simulink model "model"  (R2023b)
settings: Solver=VariableStepAuto  StartTime=0.0  StopTime=10.0  RelTol=1e-3
undefined symbols (not defined in the file): DiscIntNeverNeededParam, Newton, Raphson
libraries: simulink x43, slpidlib x11
(part 2 of 2)

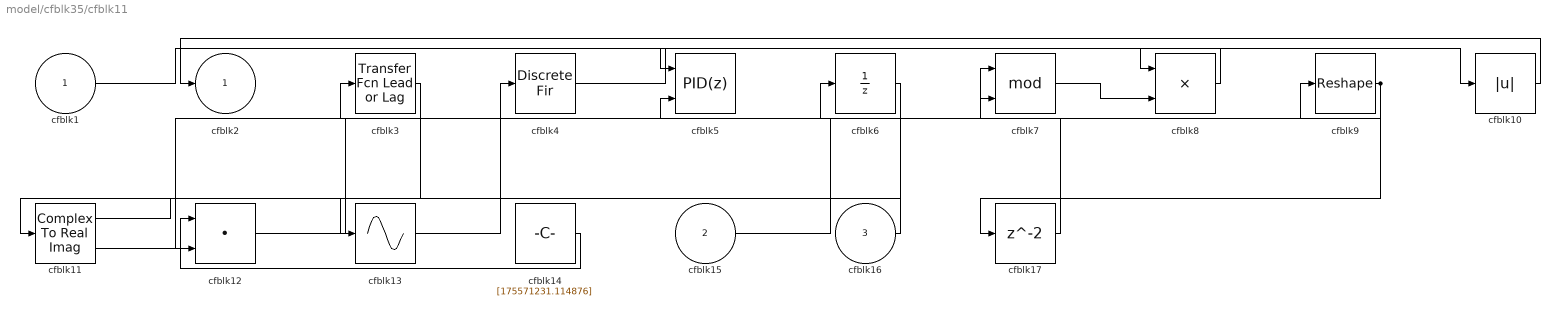
== system model/cfblk35/cfblk11 ==
  cfblk1 : Inport
  cfblk15 : Inport  Port=2
  cfblk16 : Inport  Port=3
  cfblk10 : Abs  SaturateOnIntegerOverflow=off
  cfblk11 : ComplexToRealImag
  cfblk12 : DotProduct  OutDataTypeStr=Inherit: Inherit via internal rule
  cfblk13 : Sin  TimeSource=Use external signal  SampleTime=0
  cfblk14 : Constant  Value=[175571231.114876]  SampleTime=1
  cfblk17 : Delay  SampleTime=1
  cfblk3 : simulink/Discrete/Transfer Fcn Lead or Lag  PoleZ=0.95  ZeroZ=0.75  ICPrevOutput=0.0  ICPrevInput=0.0  DoSatur=off
  cfblk4 : DiscreteFir  SampleTime=1
  cfblk5 : slpidlib/PID Controller (2DOF)  Controller=PID  Form=Parallel  TimeDomain=Discrete-time  UseExternalTs=off  SampleTime=1  IntegratorMethod=Forward Euler  FilterMethod=Forward Euler  ControllerParametersSource=internal  P=1  I=1  UseKiTs=off  D=0  N=100  UseFilter=on  b=1  c=1  TunerSelectOption=Transfer Function Based (PID Tuner App)  InitialConditionSource=internal  InitialConditionForIntegrator=0  InitialConditionForFilter=0  DifferentiatorICPrevScaledInput=0  ExternalReset=none  TrackingMode=off  Kt=1  LimitOutput=off  SatLimitsSource=internal  UpperSaturationLimit=inf  LowerSaturationLimit=-inf  LinearizeAsGain=off  AntiWindupMode=none  Kb=1  LimitIntegrator=off  UpperIntegratorSaturationLimit=inf  LowerIntegratorSaturationLimit=-inf  POutMin=[]  POutMax=[]  IOutMin=[]  IOutMax=[]  DOutMin=[]  DOutMax=[]  NOutMin=[]  NOutMax=[]  bOutMin=[]  bOutMax=[]  cOutMin=[]  cOutMax=[]  SumOutMin=[]  SumOutMax=[]  SaturationOutMin=[]  SaturationOutMax=[]  PParamMin=[]  PParamMax=[]  IParamMin=[]  IParamMax=[]  DParamMin=[]  DParamMax=[]  NParamMin=[]  NParamMax=[]  bParamMin=[]  bParamMax=[]  cParamMin=[]  cParamMax=[]  KbParamMin=[]  KbParamMax=[]  KtParamMin=[]  KtParamMax=[]  KbOutMin=[]  KbOutMax=[]  KtOutMin=[]  KtOutMax=[]  IntegratorOutMin=[]  IntegratorOutMax=[]  FilterOutMin=[]  FilterOutMax=[]  SumI1OutMin=[]  SumI1OutMax=[]  SumI2OutMin=[]  SumI2OutMax=[]  SumI3OutMin=[]  SumI3OutMax=[]  SumI4OutMin=[]  SumI4OutMax=[]  SumDOutMin=[]  SumDOutMax=[]  Sum1OutMin=[]  Sum1OutMax=[]  Sum2OutMin=[]  Sum2OutMax=[]  Sum3OutMin=[]  Sum3OutMax=[]  DifferentiatorOutMin=[]  DifferentiatorOutMax=[]  FilterDiffOutCoefMin=[]  FilterDiffOutCoefMax=[]  ReciprocalOutMin=[]  ReciprocalOutMax=[]  SumDenOutMin=[]  SumDenOutMax=[]  SumNumOutMin=[]  SumNumOutMax=[]  DivideOutMin=[]  DivideOutMax=[]  UdiffTsProdOutMin=[]  UdiffTsProdOutMax=[]  NTsProdOutMin=[]  NTsProdOutMax=[]  UintegralTsProdOutMin=[]  UintegralTsProdOutMax=[]  UngainTsProdOutMin=[]  UngainTsProdOutMax=[]  ClampingZeroOutDataTypeStr=Inherit: Inherit via back propagation  ClampingZeroOutMin=[]  ClampingZeroOutMax=[]  FilterDenConstantOutDataTypeStr=Inherit: Inherit via back propagation  FilterDenConstantOutMin=[]  FilterDenConstantOutMax=[]  PCopyOutDataTypeStr=Inherit: Inherit via back propagation  PCopyOutMin=[]  PCopyOutMax=[]  NCopyOutDataTypeStr=Inherit: Inherit via back propagation  NCopyOutMin=[]  NCopyOutMax=[]  IntegratorContinuousStateAttributes=''  IntegratorStateMustResolveToSignalObject=off  IntegratorRTWStateStorageClass=Auto  FilterContinuousStateAttributes=''  FilterStateMustResolveToSignalObject=off  FilterRTWStateStorageClass=Auto  ParallelPVariant=InternalParameters  IdealPVariant=Disabled  IVariant=InternalParameters  DVariant=InternalParameters  bVariant=InternalParameters  cVariant=InternalParameters  IntegratorVariant=Discrete  SatVariant=Disabled  AWVariant=Passthrough  PCopyVariant=Disabled  TRVariant=Disabled  FdbkBlocksVariant=Forward  IdealPFdbkVariant=Disabled  SatFdbkVariant=Disabled  DerivativeFilterVariant=ForwardEulerFilter  NVariant=InternalParameters  NCopyVariant=Disabled  FilterICVariant=InternalICsFilter  IntegratorICVariant=InternalICs  ExternalResetVariant=Disabled  TRSumVariant=Passthrough  SumFdbkVariant=Disabled  SumVariant=Sum_PID  TsampFilterVariant=InternalTs  TsampNgainVariant=Passthrough  TsampIntegralVariant=Disabled_SignalSpec  ExternalSaturationOutDataTypeStr=Inherit: Same as second input
      settings: LibrarySourceBlock=simulink/Discrete/Discrete PID Controller (2DOF)
  cfblk6 : UnitDelay  HasFrameUpgradeWarning=on
  cfblk7 : Math  Operator=mod
  cfblk8 : Product
  cfblk9 : Reshape
  cfblk2 : Outport
  wires:
  cfblk4/1 -> cfblk10/1
  cfblk9/1 -> cfblk5/2, cfblk17/1
  cfblk12/1 -> cfblk9/1
  cfblk16/1 -> cfblk6/1
  cfblk10/1 -> cfblk2/1
  cfblk14/1 -> cfblk12/1
  cfblk11/1 -> cfblk13/1
  cfblk3/1 -> cfblk12/2
  cfblk15/1 -> cfblk7/1
  cfblk6/1 -> cfblk11/1
  cfblk11/2 -> cfblk7/2
  cfblk1/1 -> cfblk8/1
  cfblk8/1 -> cfblk5/1
  cfblk7/1 -> cfblk8/2
  cfblk13/1 -> cfblk4/1
  cfblk17/1 -> cfblk3/1

== system model/cfblk36/cfblk10 ==
  cfblk1 : Inport
  cfblk10 : Delay  SampleTime=1
  cfblk3 : UnitDelay  HasFrameUpgradeWarning=on
  cfblk4 : DiscreteIntegrator  ICPrevOutput=DiscIntNeverNeededParam  ICPrevScaledInput=DiscIntNeverNeededParam
  cfblk5 : Polyval  Coefs=[ +2.081618890e-019, -1.441693666e-014, +4.719686976e-010, -8.536869453e-006, +1.621573104e-001, -8.087801117e+001 ]
  cfblk2 : Outport
  cfblk6 : Outport  Port=2
  cfblk7 : Outport  Port=3
  cfblk8 : Outport  Port=4
  cfblk9 : Outport  Port=5
  wires:
  cfblk1/1 -> cfblk7/1
  cfblk5/1 -> cfblk8/1, cfblk2/1, cfblk4/1, cfblk6/1
  cfblk3/1 -> cfblk9/1, cfblk5/1
  cfblk4/1 -> cfblk10/1
  cfblk10/1 -> cfblk3/1

== system model/cfblk36/cfblk11 ==
  cfblk1 : Inport
  cfblk12 : Inport  Port=2
  cfblk10 : Sqrt
  cfblk11 : Constant  Value=[-548459394.836145]  SampleTime=1
  cfblk14 : Delay  SampleTime=1
  cfblk3 : DiscreteFilter  SampleTime=1
  cfblk4 : Squeeze
  cfblk5 : simulink/Math Operations/Slider Gain  gain=1  low=0  high=2
  cfblk6 : Abs  SaturateOnIntegerOverflow=off
  cfblk7 : Product
  cfblk8 : Bias  Bias=[-249517717.832807]  SaturateOnIntegerOverflow=off
  cfblk9 : Sqrt
  cfblk2 : Outport
  cfblk13 : Outport  Port=2
  wires:
  cfblk11/1 -> cfblk8/1
  cfblk9/1 -> cfblk13/1
  cfblk3/1 -> cfblk7/1
  cfblk12/1 -> cfblk7/2
  cfblk6/1 -> cfblk5/1
  cfblk7/1 -> cfblk6/1
  cfblk10/1 -> cfblk2/1
  cfblk8/1 -> cfblk4/1
  cfblk1/1 -> cfblk10/1
  cfblk4/1 -> cfblk9/1
  cfblk5/1 -> cfblk14/1
  cfblk14/1 -> cfblk3/1

== system model/cfblk36/cfblk12 ==
  cfblk1 : Inport
  cfblk5 : Inport  Port=2
  cfblk6 : Inport  Port=3
  cfblk7 : Inport  Port=4
  cfblk8 : Inport  Port=5
  cfblk3 : ComplexToMagnitudeAngle
  cfblk4 : Sum  Inputs=|++
  cfblk2 : Outport
  wires:
  cfblk6/1 -> cfblk2/1
  cfblk5/1 -> cfblk3/1
  cfblk3/1 -> cfblk4/1
  cfblk7/1 -> cfblk4/2

== system model/cfblk37/cfblk10 ==
  cfblk1 : Inport
  cfblk13 : Inport  Port=2
  cfblk14 : Inport  Port=3
  cfblk15 : Inport  Port=4
  cfblk16 : Inport  Port=5
  cfblk10 : PermuteDimensions
  cfblk11 : Product  Inputs=*
  cfblk12 : Sum
  cfblk3 : simulink/Discrete/Tapped Delay  vinit=0.0  samptime=-1  NumDelays=1  DelayOrder=Oldest  includeCurrent=off
  cfblk4 : simulink/Discrete/Difference  ICPrevInput=0.0  OutMin=[]  OutMax=[]  OutDataTypeStr=Inherit: Inherit via back propagation  OutDataType=fixdt(1, 16)  OutScaling=2^-10  DoSatur=off
  cfblk5 : simulink/Discrete/Transfer Fcn First Order  PoleZ=0.95  ICPrevOutput=0.0  DoSatur=off
  cfblk6 : simulink/Discrete/Transfer Fcn Lead or Lag  PoleZ=0.95  ZeroZ=0.75  ICPrevOutput=0.0  ICPrevInput=0.0  DoSatur=off
  cfblk7 : Sum
  cfblk8 : Sum  Inputs=+-
  cfblk9 : simulink/Math Operations/Slider Gain  gain=1  low=0  high=2
  cfblk2 : Outport
  wires:
  cfblk15/1 -> cfblk5/1
  cfblk5/1 -> cfblk12/1
  cfblk4/1 -> cfblk2/1
  cfblk7/1 -> cfblk6/1
  cfblk13/1 -> cfblk7/1
  cfblk6/1 -> cfblk11/1
  cfblk11/1 -> cfblk3/1
  cfblk10/1 -> cfblk9/1
  cfblk9/1 -> cfblk7/2
  cfblk14/1 -> cfblk12/2
  cfblk12/1 -> cfblk10/1
  cfblk1/1 -> cfblk4/1
  cfblk16/1 -> cfblk8/1
  cfblk3/1 -> cfblk8/2

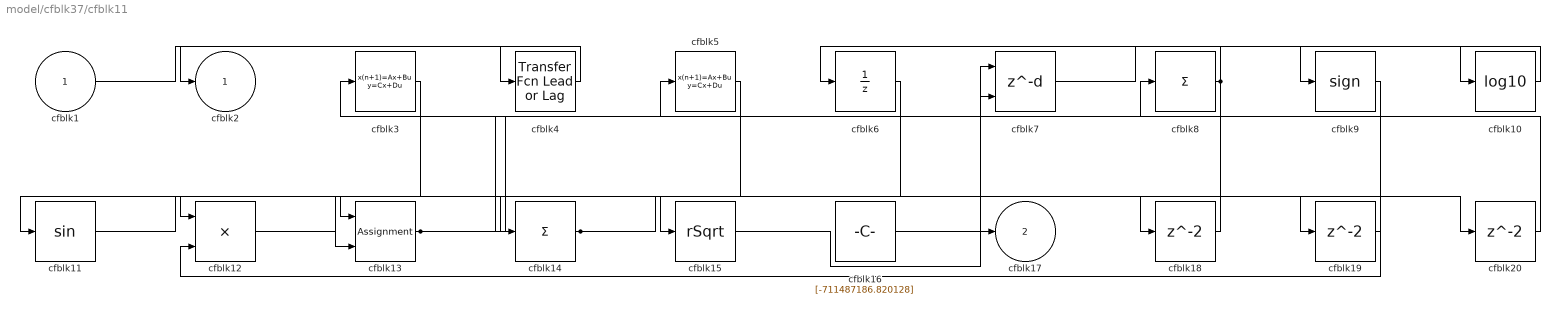
== system model/cfblk37/cfblk11 ==
  cfblk1 : Inport
  cfblk10 : Math  Operator=log10
  cfblk11 : Trigonometry
  cfblk12 : Product  Inputs=**
  cfblk13 : Assignment  DiagnosticForDimensions=Warning  IndexOptions=Index vector (dialog)  Indices=1  OutputSizes=1
  cfblk14 : Sum  Inputs=+
  cfblk15 : Sqrt  Operator=rSqrt  AlgorithmType=Newton-Raphson
  cfblk16 : Constant  Value=[-711487186.820128]  SampleTime=1
  cfblk18 : Delay  SampleTime=1
  cfblk19 : Delay  SampleTime=1
  cfblk20 : Delay  SampleTime=1
  cfblk3 : DiscreteStateSpace
  cfblk4 : simulink/Discrete/Transfer Fcn Lead or Lag  PoleZ=0.95  ZeroZ=0.75  ICPrevOutput=0.0  ICPrevInput=0.0  DoSatur=off
  cfblk5 : DiscreteStateSpace
  cfblk6 : UnitDelay  HasFrameUpgradeWarning=on
  cfblk7 : Delay  DelayLengthSource=Input port  SampleTime=1
      settings: InputPortMap=u0,p1
  cfblk8 : Sum  Inputs=+
  cfblk9 : Signum
  cfblk2 : Outport
  cfblk17 : Outport  Port=2
  wires:
  cfblk4/1 -> cfblk2/1
  cfblk6/1 -> cfblk11/1
  cfblk14/1 -> cfblk18/1, cfblk19/1
  cfblk15/1 -> cfblk7/1
  cfblk10/1 -> cfblk9/1
  cfblk16/1 -> cfblk17/1
  cfblk5/1 -> cfblk12/1
  cfblk9/1 -> cfblk12/2
  cfblk11/1 -> cfblk15/1
  cfblk1/1 -> cfblk4/1
  cfblk13/1 -> cfblk8/1, cfblk5/1
  cfblk8/1 -> cfblk14/1, cfblk6/1
  cfblk7/1 -> cfblk10/1
  cfblk3/1 -> cfblk13/2
  cfblk18/1 -> cfblk13/1
  cfblk19/1 -> cfblk3/1
  cfblk12/1 -> cfblk20/1
  cfblk20/1 -> cfblk7/2

== system model/cfblk37/cfblk12 ==
  cfblk1 : Inport
  cfblk16 : Inport  Port=2
  cfblk10 : Delay  SampleTime=1
  cfblk11 : DiscreteZeroPole  Poles=[0 0.5]  Gain=1
  cfblk12 : Sum  Inputs=-+
  cfblk13 : Sqrt  Operator=rSqrt  AlgorithmType=Newton-Raphson
  cfblk14 : UnaryMinus
  cfblk15 : Constant  Value=[60376909.899048]  SampleTime=1
  cfblk3 : simulink/Discrete/Tapped Delay  vinit=0.0  samptime=-1  NumDelays=1  DelayOrder=Oldest  includeCurrent=off
  cfblk4 : DiscreteStateSpace
  cfblk5 : UnitDelay  HasFrameUpgradeWarning=on
  cfblk6 : Delay  DelayLengthSource=Input port  SampleTime=1
      settings: InputPortMap=u0,p1
  cfblk7 : simulink/Discrete/Tapped Delay  vinit=0.0  samptime=-1  NumDelays=1  DelayOrder=Oldest  includeCurrent=off
  cfblk8 : DiscreteFir  SampleTime=1
  cfblk9 : DiscreteFir  SampleTime=1
  cfblk2 : Outport
  wires:
  cfblk10/1 -> cfblk9/1
  cfblk14/1 -> cfblk11/1
  cfblk7/1 -> cfblk14/1
  cfblk11/1 -> cfblk6/1
  cfblk1/1 -> cfblk3/1
  cfblk15/1 -> cfblk7/1
  cfblk6/1 -> cfblk5/1
  cfblk5/1 -> cfblk8/1
  cfblk16/1 -> cfblk13/1
  cfblk4/1 -> cfblk2/1
  cfblk9/1 -> cfblk12/1
  cfblk12/1 -> cfblk4/1
  cfblk8/1 -> cfblk12/2
  cfblk3/1 -> cfblk10/1
  cfblk13/1 -> cfblk6/2

== system model/cfblk37/cfblk13 ==
  cfblk1 : Inport
  cfblk11 : Inport  Port=2
  cfblk12 : Inport  Port=3
  cfblk13 : Inport  Port=4
  cfblk10 : Constant  Value=[801323161.151819]  SampleTime=1
  cfblk15 : Delay  SampleTime=1
  cfblk3 : PropagationDelay  SampleTime=1
  cfblk4 : Delay  ShowEnablePort=on  SampleTime=1
      settings: InputPortMap=u0,e6
  cfblk5 : simulink/Discrete/Transfer Fcn First Order  PoleZ=0.95  ICPrevOutput=0.0  DoSatur=off
  cfblk6 : UnitDelay  HasFrameUpgradeWarning=on
  cfblk7 : Signum
  cfblk8 : Squeeze
  cfblk9 : Sqrt  Operator=rSqrt  AlgorithmType=Newton-Raphson
  cfblk2 : Outport
  cfblk14 : Outport  Port=2
  wires:
  cfblk1/1 -> cfblk9/1
  cfblk3/1 -> cfblk7/1
  cfblk8/1 -> cfblk6/1
  cfblk10/1 -> cfblk4/1
  cfblk7/1 -> cfblk8/1
  cfblk4/1 -> cfblk2/1
  cfblk12/1 -> cfblk14/1
  cfblk11/1 -> cfblk5/1
  cfblk13/1 -> cfblk4/2
  cfblk9/1 -> cfblk3/1
  cfblk6/1 -> cfblk15/1
  cfblk15/1 -> cfblk3/2

== system model/cfblk37/cfblk8 ==
  cfblk1 : Inport
  cfblk9 : Inport  Port=2
  cfblk10 : Inport  Port=3
  cfblk11 : Delay  SampleTime=1
  cfblk3 : Delay  SampleTime=1
  cfblk4 : Product  Inputs=**
  cfblk5 : ComplexToMagnitudeAngle
  cfblk6 : Bias  Bias=[-189507740.076034]  SaturateOnIntegerOverflow=off
  cfblk7 : Squeeze
  cfblk8 : Constant  Value=[-524057900.089816]  SampleTime=1
  cfblk2 : Outport
  wires:
  cfblk4/1 -> cfblk7/1
  cfblk10/1 -> cfblk4/1
  cfblk9/1 -> cfblk6/1
  cfblk8/1 -> cfblk2/1
  cfblk6/1 -> cfblk5/1
  cfblk3/1 -> cfblk4/2
  cfblk7/1 -> cfblk11/1
  cfblk11/1 -> cfblk3/1

== system model/cfblk37/cfblk9 ==
  cfblk1 : Inport
  cfblk8 : Inport  Port=2
  cfblk9 : Inport  Port=3
  cfblk10 : Inport  Port=4
  cfblk11 : Inport  Port=5
  cfblk3 : DiscreteIntegrator  ICPrevOutput=DiscIntNeverNeededParam  ICPrevScaledInput=DiscIntNeverNeededParam
  cfblk4 : Product
  cfblk5 : Product  Inputs=*
  cfblk6 : Bias  Bias=[-689175598.464851]  SaturateOnIntegerOverflow=off
  cfblk7 : Sin  TimeSource=Use external signal  SampleTime=0
  cfblk2 : Outport
  cfblk12 : Outport  Port=2
  wires:
  cfblk9/1 -> cfblk3/1
  cfblk8/1 -> cfblk4/1
  cfblk5/1 -> cfblk6/1
  cfblk1/1 -> cfblk7/1
  cfblk11/1 -> cfblk4/2
  cfblk10/1 -> cfblk5/1
  cfblk4/1 -> cfblk2/1
  cfblk3/1 -> cfblk12/1

== system model/cfblk38/cfblk10 ==
  cfblk1 : Inport
  cfblk12 : Inport  Port=2
  cfblk13 : Inport  Port=3
  cfblk10 : MinMax  Inputs=2
  cfblk11 : Constant  Value=[-818087666.573941]  SampleTime=1
  cfblk3 : UnitDelay  HasFrameUpgradeWarning=on
  cfblk4 : Gain  Gain=[-630137339.256016]
  cfblk5 : Sum  Inputs=+
  cfblk6 : Sum  Inputs=+
  cfblk7 : Product  Inputs=*
  cfblk8 : Abs  SaturateOnIntegerOverflow=off
  cfblk9 : Reshape
  cfblk2 : Outport
  cfblk14 : Outport  Port=2
  wires:
  cfblk10/1 -> cfblk3/1
  cfblk3/1 -> cfblk8/1
  cfblk1/1 -> cfblk9/1
  cfblk8/1 -> cfblk5/1
  cfblk9/1 -> cfblk10/1
  cfblk11/1 -> cfblk6/1
  cfblk6/1 -> cfblk4/1
  cfblk4/1 -> cfblk10/2
  cfblk12/1 -> cfblk14/1
  cfblk5/1 -> cfblk7/1
  cfblk13/1 -> cfblk2/1

== system model/cfblk38/cfblk11 ==
  cfblk1 : Inport
  cfblk7 : Inport  Port=2
  cfblk3 : Delay  SampleTime=1
  cfblk4 : Delay  SampleTime=1
  cfblk5 : DiscreteFilter  SampleTime=1
  cfblk6 : Constant  Value=[-364935812.743680]  SampleTime=1
  cfblk2 : Outport
  cfblk8 : Outport  Port=2
  cfblk9 : Outport  Port=3
  wires:
  cfblk3/1 -> cfblk8/1
  cfblk1/1 -> cfblk5/1
  cfblk6/1 -> cfblk2/1
  cfblk5/1 -> cfblk4/1
  cfblk7/1 -> cfblk3/1
  cfblk4/1 -> cfblk9/1

== system model/cfblk38/cfblk12 ==
  cfblk1 : Inport
  cfblk3 : simulink/Discrete/Tapped Delay  vinit=0.0  samptime=-1  NumDelays=1  DelayOrder=Oldest  includeCurrent=off
  cfblk4 : Delay  ShowEnablePort=on  SampleTime=1
      settings: InputPortMap=u0,e6
  cfblk5 : DiscreteStateSpace
  cfblk6 : Gain  Gain=[600080903.886749]
  cfblk7 : Constant  Value=[-234072061.561648]  SampleTime=1
  cfblk8 : Constant  Value=[261940061.703511]  SampleTime=1
  cfblk2 : Outport
  wires:
  cfblk3/1 -> cfblk4/1
  cfblk7/1 -> cfblk3/1
  cfblk1/1 -> cfblk6/1
  cfblk5/1 -> cfblk4/2
  cfblk4/1 -> cfblk2/1
  cfblk6/1 -> cfblk5/1

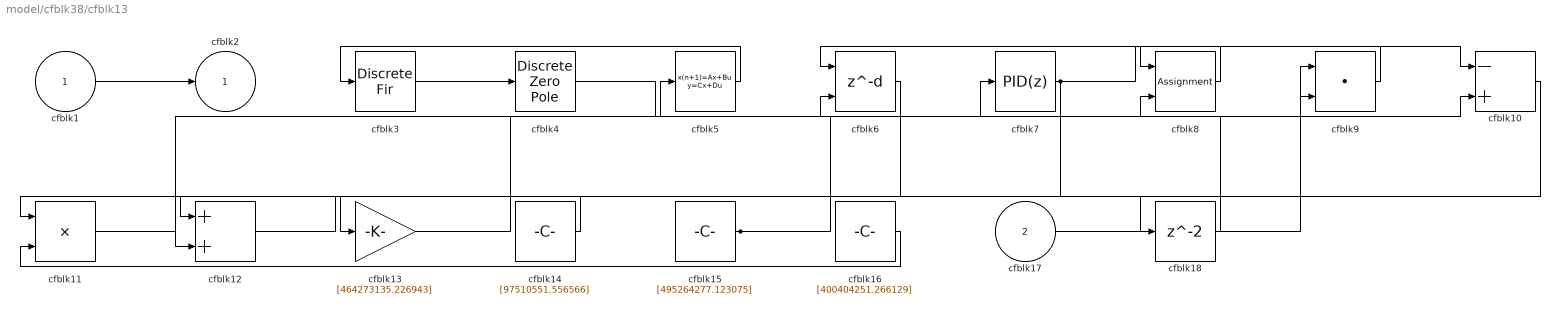
== system model/cfblk38/cfblk13 ==
  cfblk1 : Inport
  cfblk17 : Inport  Port=2
  cfblk10 : Sum  Inputs=-+
  cfblk11 : Product
  cfblk12 : Sum
  cfblk13 : Gain  Gain=[464273135.226943]
  cfblk14 : Constant  Value=[97510551.556566]  SampleTime=1
  cfblk15 : Constant  Value=[495264277.123075]  SampleTime=1
  cfblk16 : Constant  Value=[400404251.266129]  SampleTime=1
  cfblk18 : Delay  SampleTime=1
  cfblk3 : DiscreteFir  SampleTime=1
  cfblk4 : DiscreteZeroPole  Poles=[0 0.5]  Gain=1
  cfblk5 : DiscreteStateSpace
  cfblk6 : Delay  DelayLengthSource=Input port  SampleTime=1
      settings: InputPortMap=u0,p1
  cfblk7 : slpidlib/PID Controller  Controller=PID  Form=Parallel  TimeDomain=Discrete-time  UseExternalTs=off  SampleTime=1  IntegratorMethod=Forward Euler  FilterMethod=Forward Euler  ControllerParametersSource=internal  P=1  I=1  UseKiTs=off  D=0  N=100  UseFilter=on  TunerSelectOption=Transfer Function Based (PID Tuner App)  InitialConditionSource=internal  InitialConditionForIntegrator=0  InitialConditionForFilter=0  DifferentiatorICPrevScaledInput=0  ExternalReset=none  TrackingMode=off  Kt=1  LimitOutput=off  SatLimitsSource=internal  UpperSaturationLimit=inf  LowerSaturationLimit=-inf  LinearizeAsGain=off  AntiWindupMode=none  Kb=1  LimitIntegrator=off  UpperIntegratorSaturationLimit=inf  LowerIntegratorSaturationLimit=-inf  POutMin=[]  POutMax=[]  IOutMin=[]  IOutMax=[]  DOutMin=[]  DOutMax=[]  NOutMin=[]  NOutMax=[]  SumOutMin=[]  SumOutMax=[]  SaturationOutMin=[]  SaturationOutMax=[]  PParamMin=[]  PParamMax=[]  IParamMin=[]  IParamMax=[]  DParamMin=[]  DParamMax=[]  NParamMin=[]  NParamMax=[]  KbParamMin=[]  KbParamMax=[]  KtParamMin=[]  KtParamMax=[]  KbOutMin=[]  KbOutMax=[]  KtOutMin=[]  KtOutMax=[]  IntegratorOutMin=[]  IntegratorOutMax=[]  FilterOutMin=[]  FilterOutMax=[]  SumI1OutMin=[]  SumI1OutMax=[]  SumI2OutMin=[]  SumI2OutMax=[]  SumI3OutMin=[]  SumI3OutMax=[]  SumI4OutMin=[]  SumI4OutMax=[]  SumDOutMin=[]  SumDOutMax=[]  DifferentiatorOutMin=[]  DifferentiatorOutMax=[]  FilterDiffOutCoefMin=[]  FilterDiffOutCoefMax=[]  ReciprocalOutMin=[]  ReciprocalOutMax=[]  SumDenOutMin=[]  SumDenOutMax=[]  SumNumOutMin=[]  SumNumOutMax=[]  DivideOutMin=[]  DivideOutMax=[]  UdiffTsProdOutMin=[]  UdiffTsProdOutMax=[]  NTsProdOutMin=[]  NTsProdOutMax=[]  UintegralTsProdOutMin=[]  UintegralTsProdOutMax=[]  UngainTsProdOutMin=[]  UngainTsProdOutMax=[]  ClampingZeroOutDataTypeStr=Inherit: Inherit via back propagation  ClampingZeroOutMin=[]  ClampingZeroOutMax=[]  FilterDenConstantOutDataTypeStr=Inherit: Inherit via back propagation  FilterDenConstantOutMin=[]  FilterDenConstantOutMax=[]  PCopyOutDataTypeStr=Inherit: Inherit via back propagation  PCopyOutMin=[]  PCopyOutMax=[]  NCopyOutDataTypeStr=Inherit: Inherit via back propagation  NCopyOutMin=[]  NCopyOutMax=[]  IntegratorContinuousStateAttributes=''  IntegratorStateMustResolveToSignalObject=off  IntegratorRTWStateStorageClass=Auto  FilterContinuousStateAttributes=''  FilterStateMustResolveToSignalObject=off  FilterRTWStateStorageClass=Auto  ParallelPVariant=InternalParameters  IdealPVariant=Disabled  IVariant=InternalParameters  DVariant=InternalParameters  IntegratorVariant=Discrete  SatVariant=Disabled  AWVariant=Passthrough  PCopyVariant=Disabled  TRVariant=Disabled  FdbkBlocksVariant=Forward  IdealPFdbkVariant=Disabled  SatFdbkVariant=Disabled  DerivativeFilterVariant=ForwardEulerFilter  NVariant=InternalParameters  NCopyVariant=Disabled  FilterICVariant=InternalICsFilter  IntegratorICVariant=InternalICs  ExternalResetVariant=Disabled  TRSumVariant=Passthrough  SumFdbkVariant=Disabled  SumVariant=Sum_PID  TsampFilterVariant=InternalTs  TsampNgainVariant=Passthrough  TsampIntegralVariant=Disabled_SignalSpec  ExternalSaturationOutDataTypeStr=Inherit: Same as second input
      settings: LibrarySourceBlock=simulink/Discrete/Discrete PID Controller
  cfblk8 : Assignment  DiagnosticForDimensions=Warning  IndexOptions=Index vector (dialog)  Indices=1  OutputSizes=1
  cfblk9 : DotProduct  OutDataTypeStr=Inherit: Inherit via internal rule
  cfblk2 : Outport
  wires:
  cfblk1/1 -> cfblk2/1
  cfblk10/1 -> cfblk11/1
  cfblk16/1 -> cfblk11/2
  cfblk14/1 -> cfblk13/1
  cfblk3/1 -> cfblk4/1
  cfblk9/1 -> cfblk8/1
  cfblk6/1 -> cfblk12/1
  cfblk5/1 -> cfblk3/1
  cfblk13/1 -> cfblk5/1
  cfblk17/1 -> cfblk9/1
  cfblk15/1 -> cfblk7/1, cfblk10/2
  cfblk11/1 -> cfblk8/2
  cfblk8/1 -> cfblk6/1
  cfblk7/1 -> cfblk12/2, cfblk10/1
  cfblk4/1 -> cfblk9/2
  cfblk12/1 -> cfblk18/1
  cfblk18/1 -> cfblk6/2

== system model/cfblk38/cfblk14 ==
  cfblk1 : Inport
  cfblk14 : Inport  Port=2
  cfblk15 : Inport  Port=3
  cfblk10 : Squeeze
  cfblk11 : PermuteDimensions
  cfblk12 : Product  Inputs=*
  cfblk13 : Sqrt
  cfblk3 : UnitDelay  HasFrameUpgradeWarning=on
  cfblk4 : slpidlib/PID Controller  Controller=PID  Form=Parallel  TimeDomain=Discrete-time  UseExternalTs=off  SampleTime=1  IntegratorMethod=Forward Euler  FilterMethod=Forward Euler  ControllerParametersSource=internal  P=1  I=1  UseKiTs=off  D=0  N=100  UseFilter=on  TunerSelectOption=Transfer Function Based (PID Tuner App)  InitialConditionSource=internal  InitialConditionForIntegrator=0  InitialConditionForFilter=0  DifferentiatorICPrevScaledInput=0  ExternalReset=none  TrackingMode=off  Kt=1  LimitOutput=off  SatLimitsSource=internal  UpperSaturationLimit=inf  LowerSaturationLimit=-inf  LinearizeAsGain=off  AntiWindupMode=none  Kb=1  LimitIntegrator=off  UpperIntegratorSaturationLimit=inf  LowerIntegratorSaturationLimit=-inf  POutMin=[]  POutMax=[]  IOutMin=[]  IOutMax=[]  DOutMin=[]  DOutMax=[]  NOutMin=[]  NOutMax=[]  SumOutMin=[]  SumOutMax=[]  SaturationOutMin=[]  SaturationOutMax=[]  PParamMin=[]  PParamMax=[]  IParamMin=[]  IParamMax=[]  DParamMin=[]  DParamMax=[]  NParamMin=[]  NParamMax=[]  KbParamMin=[]  KbParamMax=[]  KtParamMin=[]  KtParamMax=[]  KbOutMin=[]  KbOutMax=[]  KtOutMin=[]  KtOutMax=[]  IntegratorOutMin=[]  IntegratorOutMax=[]  FilterOutMin=[]  FilterOutMax=[]  SumI1OutMin=[]  SumI1OutMax=[]  SumI2OutMin=[]  SumI2OutMax=[]  SumI3OutMin=[]  SumI3OutMax=[]  SumI4OutMin=[]  SumI4OutMax=[]  SumDOutMin=[]  SumDOutMax=[]  DifferentiatorOutMin=[]  DifferentiatorOutMax=[]  FilterDiffOutCoefMin=[]  FilterDiffOutCoefMax=[]  ReciprocalOutMin=[]  ReciprocalOutMax=[]  SumDenOutMin=[]  SumDenOutMax=[]  SumNumOutMin=[]  SumNumOutMax=[]  DivideOutMin=[]  DivideOutMax=[]  UdiffTsProdOutMin=[]  UdiffTsProdOutMax=[]  NTsProdOutMin=[]  NTsProdOutMax=[]  UintegralTsProdOutMin=[]  UintegralTsProdOutMax=[]  UngainTsProdOutMin=[]  UngainTsProdOutMax=[]  ClampingZeroOutDataTypeStr=Inherit: Inherit via back propagation  ClampingZeroOutMin=[]  ClampingZeroOutMax=[]  FilterDenConstantOutDataTypeStr=Inherit: Inherit via back propagation  FilterDenConstantOutMin=[]  FilterDenConstantOutMax=[]  PCopyOutDataTypeStr=Inherit: Inherit via back propagation  PCopyOutMin=[]  PCopyOutMax=[]  NCopyOutDataTypeStr=Inherit: Inherit via back propagation  NCopyOutMin=[]  NCopyOutMax=[]  IntegratorContinuousStateAttributes=''  IntegratorStateMustResolveToSignalObject=off  IntegratorRTWStateStorageClass=Auto  FilterContinuousStateAttributes=''  FilterStateMustResolveToSignalObject=off  FilterRTWStateStorageClass=Auto  ParallelPVariant=InternalParameters  IdealPVariant=Disabled  IVariant=InternalParameters  DVariant=InternalParameters  IntegratorVariant=Discrete  SatVariant=Disabled  AWVariant=Passthrough  PCopyVariant=Disabled  TRVariant=Disabled  FdbkBlocksVariant=Forward  IdealPFdbkVariant=Disabled  SatFdbkVariant=Disabled  DerivativeFilterVariant=ForwardEulerFilter  NVariant=InternalParameters  NCopyVariant=Disabled  FilterICVariant=InternalICsFilter  IntegratorICVariant=InternalICs  ExternalResetVariant=Disabled  TRSumVariant=Passthrough  SumFdbkVariant=Disabled  SumVariant=Sum_PID  TsampFilterVariant=InternalTs  TsampNgainVariant=Passthrough  TsampIntegralVariant=Disabled_SignalSpec  ExternalSaturationOutDataTypeStr=Inherit: Same as second input
      settings: LibrarySourceBlock=simulink/Discrete/Discrete PID Controller
  cfblk5 : simulink/Discrete/Tapped Delay  vinit=0.0  samptime=-1  NumDelays=1  DelayOrder=Oldest  includeCurrent=off
  cfblk6 : Sqrt
  cfblk7 : Assignment  DiagnosticForDimensions=Warning  IndexOptions=Index vector (dialog)  Indices=1  OutputSizes=1
  cfblk8 : Sin  TimeSource=Use external signal  SampleTime=0
  cfblk9 : Sin  TimeSource=Use external signal  SampleTime=0
  cfblk2 : Outport
  wires:
  cfblk4/1 -> cfblk12/1
  cfblk6/1 -> cfblk3/1
  cfblk1/1 -> cfblk5/1
  cfblk10/1 -> cfblk9/1
  cfblk11/1 -> cfblk10/1
  cfblk13/1 -> cfblk2/1
  cfblk15/1 -> cfblk4/1
  cfblk3/1 -> cfblk8/1
  cfblk5/1 -> cfblk6/1
  cfblk9/1 -> cfblk7/1
  cfblk14/1 -> cfblk11/1
  cfblk12/1 -> cfblk7/2
  cfblk7/1 -> cfblk13/1

== system model/cfblk38/cfblk8 ==
  cfblk1 : Inport
  cfblk9 : Inport  Port=2
  cfblk3 : Gain  Gain=[-893617306.951323]
  cfblk4 : Product
  cfblk5 : Sum  Inputs=+
  cfblk6 : Reshape
  cfblk7 : Trigonometry
  cfblk8 : Constant  Value=[719142667.653618]  SampleTime=1
  cfblk2 : Outport
  cfblk10 : Outport  Port=2
  cfblk11 : Outport  Port=3
  wires:
  cfblk5/1 -> cfblk3/1
  cfblk3/1 -> cfblk11/1
  cfblk8/1 -> cfblk4/1, cfblk7/1
  cfblk6/1 -> cfblk2/1
  cfblk9/1 -> cfblk4/2
  cfblk4/1 -> cfblk10/1
  cfblk1/1 -> cfblk5/1
  cfblk7/1 -> cfblk6/1

== system model/cfblk38/cfblk9 ==
  cfblk1 : Inport
  cfblk7 : Inport  Port=2
  cfblk8 : Inport  Port=3
  cfblk3 : DiscreteTransferFcn  SampleTime=1
  cfblk4 : UnaryMinus
  cfblk5 : UnaryMinus
  cfblk6 : Constant  Value=[970426307.203716]  SampleTime=1
  cfblk2 : Outport
  cfblk9 : Outport  Port=2
  cfblk10 : Outport  Port=3
  wires:
  cfblk5/1 -> cfblk2/1
  cfblk1/1 -> cfblk4/1
  cfblk7/1 -> cfblk3/1
  cfblk3/1 -> cfblk9/1
  cfblk6/1 -> cfblk5/1
  cfblk4/1 -> cfblk10/1

== system model/cfblk39/cfblk10 ==
  cfblk1 : Inport
  cfblk11 : Inport  Port=2
  cfblk12 : Inport  Port=3
  cfblk10 : Constant  Value=[-430199746.707510]  SampleTime=1
  cfblk3 : Delay  DelayLengthSource=Input port  SampleTime=1
      settings: InputPortMap=u0,p1
  cfblk4 : Sin  TimeSource=Use external signal  SampleTime=0
  cfblk5 : Sum  Inputs=+
  cfblk6 : PermuteDimensions
  cfblk7 : Sum  Inputs=|++
  cfblk8 : Product  Inputs=**
  cfblk9 : Sum  Inputs=+-
  cfblk2 : Outport
  cfblk13 : Outport  Port=2
  wires:
  cfblk10/1 -> cfblk6/1
  cfblk3/1 -> cfblk8/1
  cfblk5/1 -> cfblk4/1
  cfblk6/1 -> cfblk7/1, cfblk3/2
  cfblk8/1 -> cfblk13/1
  cfblk4/1 -> cfblk8/2
  cfblk1/1 -> cfblk7/2
  cfblk12/1 -> cfblk2/1, cfblk9/2
  cfblk11/1 -> cfblk5/1
  cfblk7/1 -> cfblk9/1
  cfblk9/1 -> cfblk3/1

== system model/cfblk39/cfblk11 ==
  cfblk1 : Inport
  cfblk9 : Inport  Port=2
  cfblk10 : Inport  Port=3
  cfblk11 : Inport  Port=4
  cfblk12 : Inport  Port=5
  cfblk3 : DiscreteStateSpace
  cfblk4 : DiscreteIntegrator  ICPrevOutput=DiscIntNeverNeededParam  ICPrevScaledInput=DiscIntNeverNeededParam
  cfblk5 : Sin  TimeSource=Use external signal  SampleTime=0
  cfblk6 : DotProduct  OutDataTypeStr=Inherit: Inherit via internal rule
  cfblk7 : Constant  Value=[-722446577.434283]  SampleTime=1
  cfblk8 : Constant  Value=[-47518749.440726]  SampleTime=1
  cfblk2 : Outport
  cfblk13 : Outport  Port=2
  cfblk14 : Outport  Port=3
  wires:
  cfblk9/1 -> cfblk6/1
  cfblk5/1 -> cfblk14/1
  cfblk11/1 -> cfblk4/1
  cfblk1/1 -> cfblk2/1
  cfblk10/1 -> cfblk6/2
  cfblk8/1 -> cfblk3/1
  cfblk7/1 -> cfblk5/1
  cfblk3/1 -> cfblk13/1

== system model/cfblk39/cfblk12 ==
  cfblk1 : Inport
  cfblk10 : Inport  Port=2
  cfblk11 : Inport  Port=3
  cfblk12 : Inport  Port=4
  cfblk14 : Delay  SampleTime=1
  cfblk3 : simulink/Discrete/Difference  ICPrevInput=0.0  OutMin=[]  OutMax=[]  OutDataTypeStr=Inherit: Inherit via back propagation  OutDataType=fixdt(1, 16)  OutScaling=2^-10  DoSatur=off
  cfblk4 : DiscreteZeroPole  Poles=[0 0.5]  Gain=1
  cfblk5 : Delay  ShowEnablePort=on  SampleTime=1
      settings: InputPortMap=u0,e6
  cfblk6 : Gain  Gain=[-375453854.574921]
  cfblk7 : Abs  SaturateOnIntegerOverflow=off
  cfblk8 : Constant  Value=[309716630.147981]  SampleTime=1
  cfblk9 : Constant  Value=[-168676981.693167]  SampleTime=1
  cfblk2 : Outport
  cfblk13 : Outport  Port=2
  wires:
  cfblk1/1 -> cfblk13/1
  cfblk8/1 -> cfblk4/1
  cfblk5/1 -> cfblk6/1
  cfblk10/1 -> cfblk7/1
  cfblk11/1 -> cfblk2/1
  cfblk7/1 -> cfblk5/1
  cfblk3/1 -> cfblk5/2
  cfblk6/1 -> cfblk14/1
  cfblk14/1 -> cfblk3/1

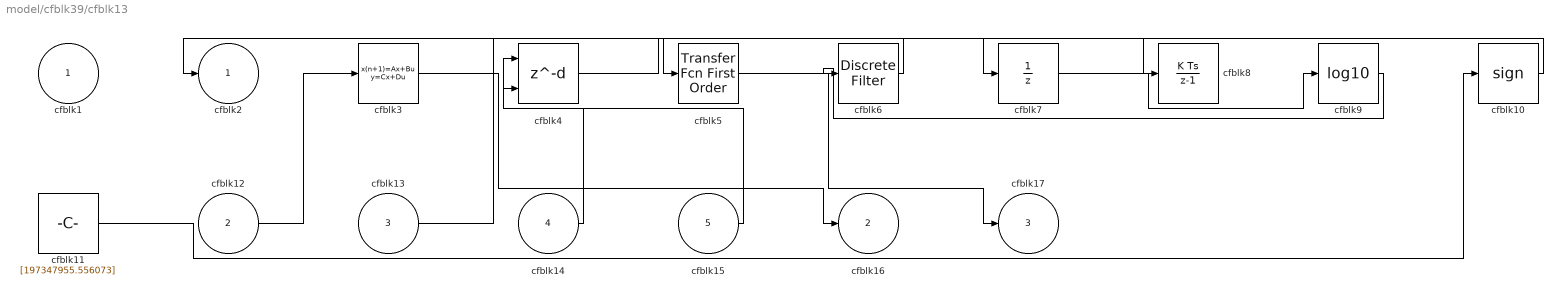
== system model/cfblk39/cfblk13 ==
  cfblk1 : Inport
  cfblk12 : Inport  Port=2
  cfblk13 : Inport  Port=3
  cfblk14 : Inport  Port=4
  cfblk15 : Inport  Port=5
  cfblk10 : Signum
  cfblk11 : Constant  Value=[197347955.556073]  SampleTime=1
  cfblk3 : DiscreteStateSpace
  cfblk4 : Delay  DelayLengthSource=Input port  SampleTime=1
      settings: InputPortMap=u0,p1
  cfblk5 : simulink/Discrete/Transfer Fcn First Order  PoleZ=0.95  ICPrevOutput=0.0  DoSatur=off
  cfblk6 : DiscreteFilter  SampleTime=1
  cfblk7 : UnitDelay  HasFrameUpgradeWarning=on
  cfblk8 : DiscreteIntegrator  ICPrevOutput=DiscIntNeverNeededParam  ICPrevScaledInput=DiscIntNeverNeededParam
  cfblk9 : Math  Operator=log10
  cfblk2 : Outport
  cfblk16 : Outport  Port=2
  cfblk17 : Outport  Port=3
  wires:
  cfblk12/1 -> cfblk3/1
  cfblk15/1 -> cfblk4/1
  cfblk5/1 -> cfblk17/1
  cfblk14/1 -> cfblk4/2
  cfblk10/1 -> cfblk7/1
  cfblk7/1 -> cfblk9/1
  cfblk13/1 -> cfblk5/1
  cfblk3/1 -> cfblk16/1
  cfblk4/1 -> cfblk8/1
  cfblk9/1 -> cfblk6/1
  cfblk6/1 -> cfblk2/1
  cfblk11/1 -> cfblk10/1

== system model/cfblk39/cfblk14 ==
  cfblk1 : Inport
  cfblk8 : Inport  Port=2
  cfblk9 : Inport  Port=3
  cfblk10 : Inport  Port=4
  cfblk3 : simulink/Discrete/Tapped Delay  vinit=0.0  samptime=-1  NumDelays=1  DelayOrder=Oldest  includeCurrent=off
  cfblk4 : Product  Inputs=**
  cfblk5 : Constant  Value=[-298102019.536058]  SampleTime=1
  cfblk6 : Constant  Value=[394898119.156315]  SampleTime=1
  cfblk7 : Constant  Value=[-946998443.364874]  SampleTime=1
  cfblk2 : Outport
  cfblk11 : Outport  Port=2
  wires:
  cfblk3/1 -> cfblk4/1
  cfblk8/1 -> cfblk2/1
  cfblk5/1 -> cfblk11/1
  cfblk1/1 -> cfblk4/2
  cfblk7/1 -> cfblk3/1

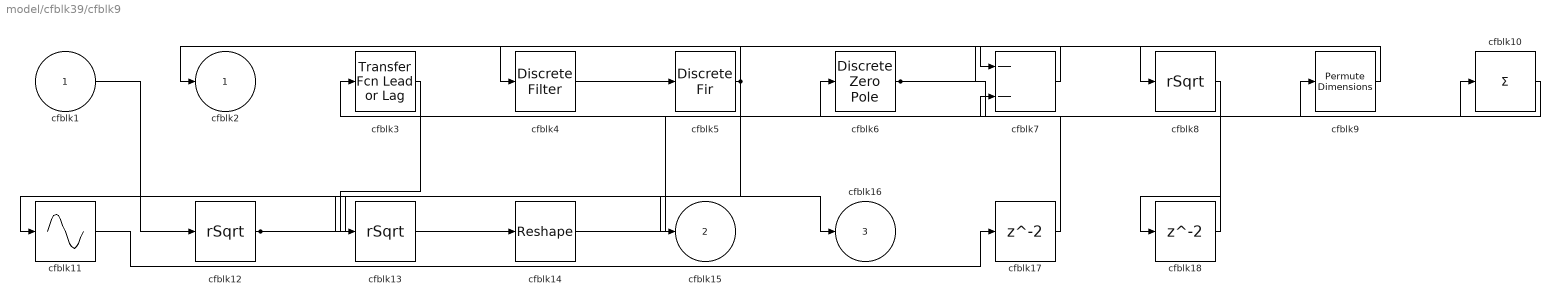
== system model/cfblk39/cfblk9 ==
  cfblk1 : Inport
  cfblk10 : Sum  Inputs=+
  cfblk11 : Sin  TimeSource=Use external signal  SampleTime=0
  cfblk12 : Sqrt  Operator=rSqrt  AlgorithmType=Newton-Raphson
  cfblk13 : Sqrt  Operator=rSqrt  AlgorithmType=Newton-Raphson
  cfblk14 : Reshape
  cfblk17 : Delay  SampleTime=1
  cfblk18 : Delay  SampleTime=1
  cfblk3 : simulink/Discrete/Transfer Fcn Lead or Lag  PoleZ=0.95  ZeroZ=0.75  ICPrevOutput=0.0  ICPrevInput=0.0  DoSatur=off
  cfblk4 : DiscreteFilter  SampleTime=1
  cfblk5 : DiscreteFir  SampleTime=1
  cfblk6 : DiscreteZeroPole  Poles=[0 0.5]  Gain=1
  cfblk7 : Sum  Inputs=--
  cfblk8 : Sqrt  Operator=rSqrt  AlgorithmType=Newton-Raphson
  cfblk9 : PermuteDimensions
  cfblk2 : Outport
  cfblk15 : Outport  Port=2
  cfblk16 : Outport  Port=3
  wires:
  cfblk9/1 -> cfblk7/1
  cfblk12/1 -> cfblk16/1, cfblk15/1
  cfblk5/1 -> cfblk2/1, cfblk11/1
  cfblk3/1 -> cfblk13/1
  cfblk13/1 -> cfblk14/1
  cfblk6/1 -> cfblk9/1, cfblk8/1
  cfblk4/1 -> cfblk5/1
  cfblk10/1 -> cfblk7/2
  cfblk1/1 -> cfblk12/1
  cfblk14/1 -> cfblk10/1
  cfblk7/1 -> cfblk4/1
  cfblk11/1 -> cfblk17/1
  cfblk17/1 -> cfblk3/1
  cfblk8/1 -> cfblk18/1
  cfblk18/1 -> cfblk6/1

== system model/cfblk40/cfblk11 ==
  cfblk1 : Inport
  Action Port : ActionPort  ActionPortLabel=if(u1 >= 0)
  cfblk10 : Constant  Value=[-596403052.275177]  SampleTime=1
  cfblk12 : Delay
  cfblk3 : DiscreteZeroPole  Poles=[0 0.5]  Gain=1  SampleTime=-1
  cfblk4 : DiscreteTransferFcn
  cfblk5 : DiscreteTransferFcn
  cfblk6 : Sum
  cfblk7 : UnaryMinus
  cfblk8 : Sum  Inputs=|++
  cfblk9 : MinMax  Function=max  Inputs=3
  cfblk2 : Outport
  cfblk11 : Outport  Port=2
  wires:
  cfblk3/1 -> cfblk9/1
  cfblk7/1 -> cfblk5/1
  cfblk5/1 -> cfblk4/1, cfblk3/1
  cfblk6/1 -> cfblk9/2, cfblk2/1
  cfblk8/1 -> cfblk6/2
  cfblk10/1 -> cfblk7/1
  cfblk4/1 -> cfblk8/1, cfblk11/1, cfblk9/3
  cfblk1/1 -> cfblk8/2
  cfblk9/1 -> cfblk12/1
  cfblk12/1 -> cfblk6/1

== system model/cfblk40/cfblk12 ==
  cfblk1 : Inport
  cfblk5 : Inport  Port=2
  Action Port : ActionPort  ActionPortLabel=else
  cfblk3 : Product  Inputs=**
  cfblk4 : Sum  Inputs=+
  cfblk2 : Outport
  cfblk6 : Outport  Port=2
  cfblk7 : Outport  Port=3
  wires:
  cfblk4/1 -> cfblk7/1, cfblk3/1
  cfblk1/1 -> cfblk4/1, cfblk3/2
  cfblk5/1 -> cfblk2/1
  cfblk3/1 -> cfblk6/1

== system model/cfblk40/cfblk6 ==
  cfblk1 : Inport
  cfblk5 : Inport  Port=2
  cfblk6 : Inport  Port=3
  cfblk3 : ComplexToMagnitudeAngle
  cfblk4 : Constant  Value=[953994063.598649]  SampleTime=1
  cfblk2 : Outport
  cfblk7 : Outport  Port=2
  cfblk8 : Outport  Port=3
  wires:
  cfblk5/1 -> cfblk3/1
  cfblk4/1 -> cfblk8/1
  cfblk1/1 -> cfblk7/1
  cfblk6/1 -> cfblk2/1

== system model/cfblk40/cfblk7 ==
  cfblk1 : Inport
  cfblk12 : Inport  Port=2
  cfblk13 : Inport  Port=3
  cfblk10 : Signum
  cfblk11 : Constant  Value=[242620350.389675]  SampleTime=1
  cfblk3 : simulink/Discrete/Transfer Fcn First Order  PoleZ=0.95  ICPrevOutput=0.0  DoSatur=off
  cfblk4 : simulink/Discrete/Transfer Fcn First Order  PoleZ=0.95  ICPrevOutput=0.0  DoSatur=off
  cfblk5 : DiscreteFilter  SampleTime=1
  cfblk6 : slpidlib/PID Controller  Controller=PID  Form=Parallel  TimeDomain=Discrete-time  UseExternalTs=off  SampleTime=1  IntegratorMethod=Forward Euler  FilterMethod=Forward Euler  ControllerParametersSource=internal  P=1  I=1  UseKiTs=off  D=0  N=100  UseFilter=on  TunerSelectOption=Transfer Function Based (PID Tuner App)  InitialConditionSource=internal  InitialConditionForIntegrator=0  InitialConditionForFilter=0  DifferentiatorICPrevScaledInput=0  ExternalReset=none  TrackingMode=off  Kt=1  LimitOutput=off  SatLimitsSource=internal  UpperSaturationLimit=inf  LowerSaturationLimit=-inf  LinearizeAsGain=off  AntiWindupMode=none  Kb=1  LimitIntegrator=off  UpperIntegratorSaturationLimit=inf  LowerIntegratorSaturationLimit=-inf  POutMin=[]  POutMax=[]  IOutMin=[]  IOutMax=[]  DOutMin=[]  DOutMax=[]  NOutMin=[]  NOutMax=[]  SumOutMin=[]  SumOutMax=[]  SaturationOutMin=[]  SaturationOutMax=[]  PParamMin=[]  PParamMax=[]  IParamMin=[]  IParamMax=[]  DParamMin=[]  DParamMax=[]  NParamMin=[]  NParamMax=[]  KbParamMin=[]  KbParamMax=[]  KtParamMin=[]  KtParamMax=[]  KbOutMin=[]  KbOutMax=[]  KtOutMin=[]  KtOutMax=[]  IntegratorOutMin=[]  IntegratorOutMax=[]  FilterOutMin=[]  FilterOutMax=[]  SumI1OutMin=[]  SumI1OutMax=[]  SumI2OutMin=[]  SumI2OutMax=[]  SumI3OutMin=[]  SumI3OutMax=[]  SumI4OutMin=[]  SumI4OutMax=[]  SumDOutMin=[]  SumDOutMax=[]  DifferentiatorOutMin=[]  DifferentiatorOutMax=[]  FilterDiffOutCoefMin=[]  FilterDiffOutCoefMax=[]  ReciprocalOutMin=[]  ReciprocalOutMax=[]  SumDenOutMin=[]  SumDenOutMax=[]  SumNumOutMin=[]  SumNumOutMax=[]  DivideOutMin=[]  DivideOutMax=[]  UdiffTsProdOutMin=[]  UdiffTsProdOutMax=[]  NTsProdOutMin=[]  NTsProdOutMax=[]  UintegralTsProdOutMin=[]  UintegralTsProdOutMax=[]  UngainTsProdOutMin=[]  UngainTsProdOutMax=[]  ClampingZeroOutDataTypeStr=Inherit: Inherit via back propagation  ClampingZeroOutMin=[]  ClampingZeroOutMax=[]  FilterDenConstantOutDataTypeStr=Inherit: Inherit via back propagation  FilterDenConstantOutMin=[]  FilterDenConstantOutMax=[]  PCopyOutDataTypeStr=Inherit: Inherit via back propagation  PCopyOutMin=[]  PCopyOutMax=[]  NCopyOutDataTypeStr=Inherit: Inherit via back propagation  NCopyOutMin=[]  NCopyOutMax=[]  IntegratorContinuousStateAttributes=''  IntegratorStateMustResolveToSignalObject=off  IntegratorRTWStateStorageClass=Auto  FilterContinuousStateAttributes=''  FilterStateMustResolveToSignalObject=off  FilterRTWStateStorageClass=Auto  ParallelPVariant=InternalParameters  IdealPVariant=Disabled  IVariant=InternalParameters  DVariant=InternalParameters  IntegratorVariant=Discrete  SatVariant=Disabled  AWVariant=Passthrough  PCopyVariant=Disabled  TRVariant=Disabled  FdbkBlocksVariant=Forward  IdealPFdbkVariant=Disabled  SatFdbkVariant=Disabled  DerivativeFilterVariant=ForwardEulerFilter  NVariant=InternalParameters  NCopyVariant=Disabled  FilterICVariant=InternalICsFilter  IntegratorICVariant=InternalICs  ExternalResetVariant=Disabled  TRSumVariant=Passthrough  SumFdbkVariant=Disabled  SumVariant=Sum_PID  TsampFilterVariant=InternalTs  TsampNgainVariant=Passthrough  TsampIntegralVariant=Disabled_SignalSpec  ExternalSaturationOutDataTypeStr=Inherit: Same as second input
      settings: LibrarySourceBlock=simulink/Discrete/Discrete PID Controller
  cfblk7 : simulink/Discrete/Transfer Fcn First Order  PoleZ=0.95  ICPrevOutput=0.0  DoSatur=off
  cfblk8 : Reshape
  cfblk9 : simulink/Math Operations/Slider Gain  gain=1  low=0  high=2
  cfblk2 : Outport
  cfblk14 : Outport  Port=2
  wires:
  cfblk7/1 -> cfblk3/1
  cfblk1/1 -> cfblk10/1
  cfblk3/1 -> cfblk6/1
  cfblk5/1 -> cfblk9/1
  cfblk12/1 -> cfblk7/1
  cfblk6/1 -> cfblk4/1
  cfblk9/1 -> cfblk14/1
  cfblk13/1 -> cfblk8/1
  cfblk10/1 -> cfblk5/1
  cfblk4/1 -> cfblk2/1

== system model/cfblk41/cfblk10 ==
  cfblk1 : Inport
  cfblk3 : simulink/Discrete/Transfer Fcn Real Zero  ZeroZ=0.75  ICPrevInput=0.0  DoSatur=off
  cfblk4 : DiscreteStateSpace
  cfblk5 : Delay  DelayLengthSource=Input port  SampleTime=1
      settings: InputPortMap=u0,p1
  cfblk6 : Abs  SaturateOnIntegerOverflow=off
  cfblk7 : UnaryMinus
  cfblk8 : Product
  cfblk9 : Delay  SampleTime=1
  cfblk2 : Outport
  wires:
  cfblk7/1 -> cfblk5/1, cfblk8/2
  cfblk1/1 -> cfblk6/1
  cfblk4/1 -> cfblk5/2
  cfblk6/1 -> cfblk7/1
  cfblk5/1 -> cfblk2/1
  cfblk8/1 -> cfblk3/1, cfblk4/1
  cfblk3/1 -> cfblk9/1
  cfblk9/1 -> cfblk8/1

== system model/cfblk41/cfblk11 ==
  cfblk1 : Inport
  cfblk8 : Inport  Port=2
  cfblk9 : Inport  Port=3
  cfblk3 : slpidlib/PID Controller (2DOF)  Controller=PID  Form=Parallel  TimeDomain=Discrete-time  UseExternalTs=off  SampleTime=1  IntegratorMethod=Forward Euler  FilterMethod=Forward Euler  ControllerParametersSource=internal  P=1  I=1  UseKiTs=off  D=0  N=100  UseFilter=on  b=1  c=1  TunerSelectOption=Transfer Function Based (PID Tuner App)  InitialConditionSource=internal  InitialConditionForIntegrator=0  InitialConditionForFilter=0  DifferentiatorICPrevScaledInput=0  ExternalReset=none  TrackingMode=off  Kt=1  LimitOutput=off  SatLimitsSource=internal  UpperSaturationLimit=inf  LowerSaturationLimit=-inf  LinearizeAsGain=off  AntiWindupMode=none  Kb=1  LimitIntegrator=off  UpperIntegratorSaturationLimit=inf  LowerIntegratorSaturationLimit=-inf  POutMin=[]  POutMax=[]  IOutMin=[]  IOutMax=[]  DOutMin=[]  DOutMax=[]  NOutMin=[]  NOutMax=[]  bOutMin=[]  bOutMax=[]  cOutMin=[]  cOutMax=[]  SumOutMin=[]  SumOutMax=[]  SaturationOutMin=[]  SaturationOutMax=[]  PParamMin=[]  PParamMax=[]  IParamMin=[]  IParamMax=[]  DParamMin=[]  DParamMax=[]  NParamMin=[]  NParamMax=[]  bParamMin=[]  bParamMax=[]  cParamMin=[]  cParamMax=[]  KbParamMin=[]  KbParamMax=[]  KtParamMin=[]  KtParamMax=[]  KbOutMin=[]  KbOutMax=[]  KtOutMin=[]  KtOutMax=[]  IntegratorOutMin=[]  IntegratorOutMax=[]  FilterOutMin=[]  FilterOutMax=[]  SumI1OutMin=[]  SumI1OutMax=[]  SumI2OutMin=[]  SumI2OutMax=[]  SumI3OutMin=[]  SumI3OutMax=[]  SumI4OutMin=[]  SumI4OutMax=[]  SumDOutMin=[]  SumDOutMax=[]  Sum1OutMin=[]  Sum1OutMax=[]  Sum2OutMin=[]  Sum2OutMax=[]  Sum3OutMin=[]  Sum3OutMax=[]  DifferentiatorOutMin=[]  DifferentiatorOutMax=[]  FilterDiffOutCoefMin=[]  FilterDiffOutCoefMax=[]  ReciprocalOutMin=[]  ReciprocalOutMax=[]  SumDenOutMin=[]  SumDenOutMax=[]  SumNumOutMin=[]  SumNumOutMax=[]  DivideOutMin=[]  DivideOutMax=[]  UdiffTsProdOutMin=[]  UdiffTsProdOutMax=[]  NTsProdOutMin=[]  NTsProdOutMax=[]  UintegralTsProdOutMin=[]  UintegralTsProdOutMax=[]  UngainTsProdOutMin=[]  UngainTsProdOutMax=[]  ClampingZeroOutDataTypeStr=Inherit: Inherit via back propagation  ClampingZeroOutMin=[]  ClampingZeroOutMax=[]  FilterDenConstantOutDataTypeStr=Inherit: Inherit via back propagation  FilterDenConstantOutMin=[]  FilterDenConstantOutMax=[]  PCopyOutDataTypeStr=Inherit: Inherit via back propagation  PCopyOutMin=[]  PCopyOutMax=[]  NCopyOutDataTypeStr=Inherit: Inherit via back propagation  NCopyOutMin=[]  NCopyOutMax=[]  IntegratorContinuousStateAttributes=''  IntegratorStateMustResolveToSignalObject=off  IntegratorRTWStateStorageClass=Auto  FilterContinuousStateAttributes=''  FilterStateMustResolveToSignalObject=off  FilterRTWStateStorageClass=Auto  ParallelPVariant=InternalParameters  IdealPVariant=Disabled  IVariant=InternalParameters  DVariant=InternalParameters  bVariant=InternalParameters  cVariant=InternalParameters  IntegratorVariant=Discrete  SatVariant=Disabled  AWVariant=Passthrough  PCopyVariant=Disabled  TRVariant=Disabled  FdbkBlocksVariant=Forward  IdealPFdbkVariant=Disabled  SatFdbkVariant=Disabled  DerivativeFilterVariant=ForwardEulerFilter  NVariant=InternalParameters  NCopyVariant=Disabled  FilterICVariant=InternalICsFilter  IntegratorICVariant=InternalICs  ExternalResetVariant=Disabled  TRSumVariant=Passthrough  SumFdbkVariant=Disabled  SumVariant=Sum_PID  TsampFilterVariant=InternalTs  TsampNgainVariant=Passthrough  TsampIntegralVariant=Disabled_SignalSpec  ExternalSaturationOutDataTypeStr=Inherit: Same as second input
      settings: LibrarySourceBlock=simulink/Discrete/Discrete PID Controller (2DOF)
  cfblk4 : Reshape
  cfblk5 : Constant  Value=[701087735.147808]  SampleTime=1
  cfblk6 : Constant  Value=[-631544403.551542]  SampleTime=1
  cfblk7 : Constant  Value=[75567617.252760]  SampleTime=1
  cfblk2 : Outport
  cfblk10 : Outport  Port=2
  cfblk11 : Outport  Port=3
  wires:
  cfblk5/1 -> cfblk11/1
  cfblk7/1 -> cfblk2/1
  cfblk6/1 -> cfblk10/1
  cfblk1/1 -> cfblk3/1
  cfblk8/1 -> cfblk4/1
  cfblk4/1 -> cfblk3/2

== system model/cfblk43/cfblk5 ==
  cfblk1 : Inport
  cfblk11 : Inport  Port=2
  cfblk10 : Constant  Value=[-994842037.182122]  SampleTime=1
  cfblk14 : Delay
  cfblk3 : DiscreteIntegrator  SampleTime=-1  ICPrevOutput=DiscIntNeverNeededParam  ICPrevScaledInput=DiscIntNeverNeededParam
  cfblk4 : DiscreteFilter
  cfblk5 : Sum  Inputs=-+
  cfblk6 : Sum
  cfblk7 : MinMax  Inputs=2
  cfblk8 : Product  Inputs=*
  cfblk9 : Constant  Value=[645096293.018452]  SampleTime=1
  cfblk2 : Outport
  cfblk12 : Outport  Port=2
  cfblk13 : Outport  Port=3
  wires:
  cfblk1/1 -> cfblk13/1, cfblk5/2
  cfblk10/1 -> cfblk12/1
  cfblk11/1 -> cfblk8/1
  cfblk3/1 -> cfblk6/1
  cfblk8/1 -> cfblk6/2
  cfblk9/1 -> cfblk4/1
  cfblk6/1 -> cfblk7/1
  cfblk4/1 -> cfblk5/1, cfblk7/2
  cfblk5/1 -> cfblk2/1
  cfblk7/1 -> cfblk14/1
  cfblk14/1 -> cfblk3/1

== system model/cfblk43/cfblk6 ==
  cfblk1 : Inport
  cfblk3 : DiscreteIntegrator  SampleTime=-1  ICPrevOutput=DiscIntNeverNeededParam  ICPrevScaledInput=DiscIntNeverNeededParam
  cfblk4 : ComplexToRealImag
  cfblk5 : Reshape
  cfblk6 : Constant  Value=[740463419.511785]  SampleTime=1
  cfblk2 : Outport
  cfblk7 : Outport  Port=2
  wires:
  cfblk6/1 -> cfblk7/1
  cfblk1/1 -> cfblk3/1
  cfblk5/1 -> cfblk2/1
  cfblk3/1 -> cfblk4/1
  cfblk4/1 -> cfblk5/1

== system model/cfblk44/cfblk8 ==
  cfblk1 : Inport
  cfblk12 : Inport  Port=2
  cfblk13 : Inport  Port=3
  cfblk14 : Inport  Port=4
  cfblk10 : Sum  Inputs=+
  cfblk11 : Constant  Value=[-684850580.819652]  SampleTime=1
  cfblk15 : Delay
  cfblk3 : DiscreteIntegrator  SampleTime=-1  ICPrevOutput=DiscIntNeverNeededParam  ICPrevScaledInput=DiscIntNeverNeededParam
  cfblk4 : Sqrt
  cfblk5 : Rounding
  cfblk6 : Sum  Inputs=+
  cfblk7 : Assignment  DiagnosticForDimensions=Warning  IndexOptions=Index vector (dialog)  Indices=1  OutputSizes=1
  cfblk8 : Sqrt  Operator=rSqrt  AlgorithmType=Newton-Raphson
  cfblk9 : Sum  Inputs=+-
  cfblk2 : Outport
  wires:
  cfblk14/1 -> cfblk8/1
  cfblk7/1 -> cfblk10/1
  cfblk5/1 -> cfblk6/1
  cfblk9/1 -> cfblk3/1
  cfblk6/1 -> cfblk7/1
  cfblk13/1 -> cfblk9/1
  cfblk4/1 -> cfblk9/2
  cfblk11/1 -> cfblk4/1
  cfblk8/1 -> cfblk5/1
  cfblk1/1 -> cfblk2/1
  cfblk10/1 -> cfblk15/1
  cfblk15/1 -> cfblk7/2
